simulink subsystem "Encoder_SubSystem"  (R2020b)
settings: Solver=VariableStepAuto  StartTime=0.0  StopTime=10.0  RelTol=1e-3
values from neighbouring files (symbols this model uses):
  Ts = 0.001    [loadParNominalHubBeam.m]
undefined symbols (not defined in the file or in its folder): sens
settings Model: Creator=umberto  LastModifiedBy=umberto

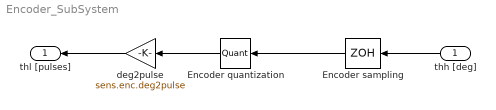
== system Encoder_SubSystem ==
  thh [deg] : Inport
  Encoder quantization : Quantizer  QuantizationInterval=360/sens.enc.ppr
  Encoder sampling : ZeroOrderHold  SampleTime=Ts
  deg2pulse : Gain  Gain=sens.enc.deg2pulse
  thl [pulses] : Outport
  wires:
  thh [deg]/1 -> Encoder sampling/1
  deg2pulse/1 -> thl [pulses]/1
  Encoder quantization/1 -> deg2pulse/1
  Encoder sampling/1 -> Encoder quantization/1
